simulink model "Linear_Simulink"  (R2025b)
settings: Solver=VariableStepAuto  StartTime=0.0  StopTime=10.0  RelTol=1e-3
undefined symbols (not defined in the file or in its folder): K, p
settings Model: Creator=chako  LastModifiedBy=chako

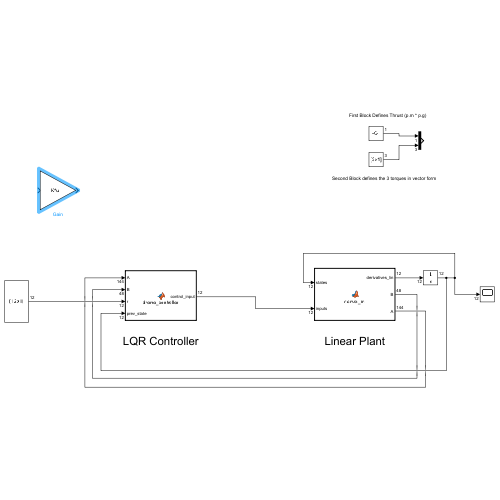
[thumbnail: Simulink's stored preview of the top-level diagram]
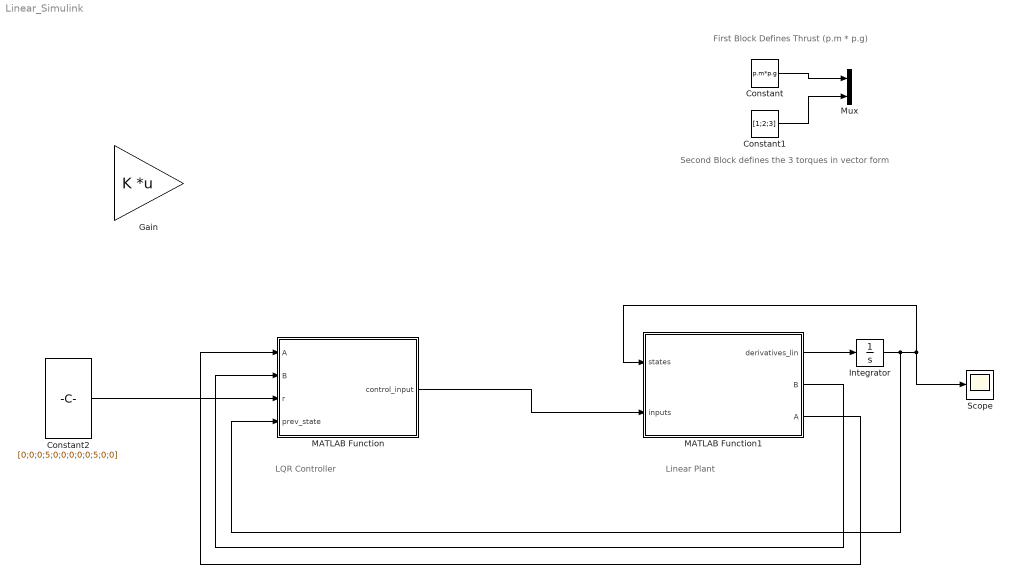
== system Linear_Simulink ==
  note: Linear Plant
  note: First Block Defines Thrust (p.m * p.g)
  note: Second Block defines the 3 torques in vector form
  note: LQR Controller
  Constant : Constant  Value=p.m*p.g
  Constant1 : Constant  Value=[1;2;3]
  Constant2 : Constant  Value=[0;0;0;5;0;0;0;0;0;5;0;0]
  Gain : Gain  Gain=K  Multiplication=Matrix(K*u)
  Integrator : Integrator
  MATLAB Function : MATLAB Function  TreatAsAtomicUnit=on
  MATLAB Function1 : MATLAB Function  TreatAsAtomicUnit=on
  Mux : Mux  Inputs=2
  Scope : Scope
  wires:
  MATLAB Function1/1(derivatives_lin) -> Integrator/1
  Constant/1 -> Mux/1
  Constant1/1 -> Mux/2
  MATLAB Function/1(control_input) -> MATLAB Function1/2(inputs)
  MATLAB Function1/3(A) -> MATLAB Function/1(A)
  MATLAB Function1/2(B) -> MATLAB Function/2(B)
  Integrator/1 -> Scope/1, MATLAB Function1/1(states), MATLAB Function/4(prev_state)
  Constant2/1 -> MATLAB Function/3(r)

== matlab function Linear_Simulink/MATLAB Function1 ==
  data: states input size=12; derivatives_lin output size=12; inputs input size=4; B output size=48; p parameter; A output size=144
function [derivatives_lin, B, A] = derive_lin(states, inputs, p)

    % Angles (roll, pitch, yaw) are small, approx 0
    % sin(x) = x, cos(x) = x 

    % Derivatives are zero
    % No torques (u2 to u4), but do need u1 = mg

    % eta is [phi, theta, psi] = roll pitch yaw
    xi= states(1:3); % x, y, z
    xid = states(4:6); %x_prime, y_prime, z_prime
    eta = states(7:9); % roll, pitch, yaw 
    etad = states(10:12); % roll_prime, pitch_prime, yaw_prime


    % Derivative of xi is xid

    % Calculative derivatives of xid
    % xidd = -(p.kD/p.m)*xid + [eta(2); -eta(1); 0]*p.g + [0;0;1]*inputs(1);
    % Calculative derivatives of etad
    % etadd = inputs
    A = [0 0 0   1 0 0           0 0 0   0 0 0;
         0 0 0   0 1 0           0 0 0   0 0 0;
         0 0 0   0 0 1           0 0 0   0 0 0;
         0 0 0   -p.kD/p.m 0 0   0 p.g 0   0 0 0;
         0 0 0   0 -p.kD/p.m 0   -p.g 0 0   0 0 0;
         0 0 0   0 0 -p.kD/p.m   0 0 0   0 0 0;
         0 0 0   0 0 0           0 0 0   1 0 0;
         0 0 0   0 0 0           0 0 0   0 1 0;
         0 0 0   0 0 0           0 0 0   0 0 1;
         0 0 0   0 0 0           0 0 0   0 0 0;
         0 0 0   0 0 0           0 0 0   0 0 0;
         0 0 0   0 0 0           0 0 0   0 0 0];

    B = [0 0 0 0;
         0 0 0 0;
         0 0 0 0;

         0 0 0 0;
         0 0 0 0;
         1/p.m 0 0 0;

         0 0 0 0;
         0 0 0 0;
         0 0 0 0;

         0 1/p.Ixx 0 0;
         0 0 1/p.Iyy 0;
         0 0 0 1/p.Izz;
         ];

    derivatives_lin = A * states + B * inputs;
end

== matlab function Linear_Simulink/MATLAB Function ==
  data: A input size=144; control_input output size=12; B input size=48; r input size=12; prev_state input size=12
function control_input = drone_controller(A, B, r, prev_state)

% Linearized Plant A, B given
error = r - prev_state;

% LQR
Q = eye(12); % Cost function weighing states
R = ones(4,1); % Cost function weighing inputs
N = 0; % Optional cross term matrix

[K, S, P] = lqr(A, B, Q, R, N);

G1sfu = ss(A-B*K,B,-K,0); % TF: Reference input to control input

t = 0; % Collecting one data point

% u1 : thurst
% u2: torque from roll
% u3: torque from pitch
% u4: torque from yaw
[control_input, tout] = lsim(G1sfu, error, t);

end
